simulink model "GolfSwing3D_InterfaceBlocks"  (R2024b)
settings: Solver=VariableStepAuto  StartTime=0.0  StopTime=StopTime  MaxStep=0.001  RelTol=1e-3
model workspace: external: MAT-File 3DModelInputs.mat (data not in the file)
undefined symbols (not defined in the file or in its folder): GripStrength, KillswitchFinalValue, KillswitchInitialValue, KillswitchStepTime, LeftLowerArmLength, PlaneTilt, RightLowerArmLength, UpperTorsoLength, X, Y, Z
libraries: nesl_utility x356, sm_lib x136, matrix_library x11, fl_lib x6, simulink x1
(part 4 of 13)

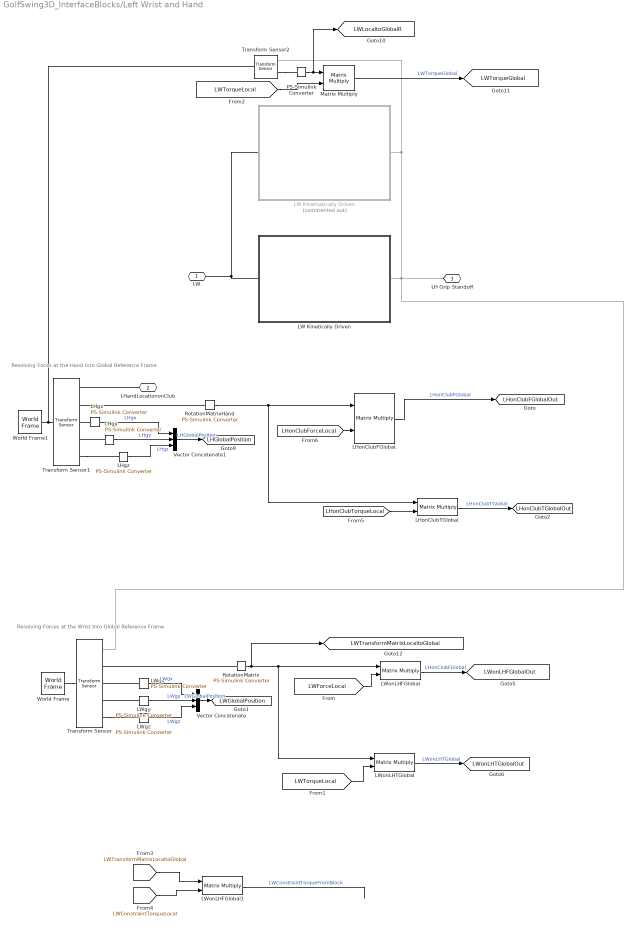
== system GolfSwing3D_InterfaceBlocks/Left Wrist and Hand ==
  note: Resolving Forces at the Wrist Into Global Reference Frame
  note: Resolving Foces at the Hand Into Global Reference Frame
  LHgx : nesl_utility/PS-Simulink Converter  PhysicalDomain=network_engine_domain  SubClassName=ps_output  LeftPortType=input  RightPortType=output  PseudoPeriodic=off  Frequencies=[]  VectorFormat=1-D array  Unit=inherit  AffineConversion=off
  LHgy : nesl_utility/PS-Simulink Converter  PhysicalDomain=network_engine_domain  SubClassName=ps_output  LeftPortType=input  RightPortType=output  PseudoPeriodic=off  Frequencies=[]  VectorFormat=1-D array  Unit=inherit  AffineConversion=off
  LHgz : nesl_utility/PS-Simulink Converter  PhysicalDomain=network_engine_domain  SubClassName=ps_output  LeftPortType=input  RightPortType=output  PseudoPeriodic=off  Frequencies=[]  VectorFormat=1-D array  Unit=inherit  AffineConversion=off
  LHonClubFGlobal. : Product  Multiplication=Matrix(*)
  LHonClubTGlobal. : Product  Multiplication=Matrix(*)
  LW Kinematically Driven : Subsystem  Commented=on
  LW Kinetically Driven : Subsystem
  LWgx : nesl_utility/PS-Simulink Converter  PhysicalDomain=network_engine_domain  SubClassName=ps_output  LeftPortType=input  RightPortType=output  PseudoPeriodic=off  Frequencies=[]  VectorFormat=1-D array  Unit=inherit  AffineConversion=off
  LWgy : nesl_utility/PS-Simulink Converter  PhysicalDomain=network_engine_domain  SubClassName=ps_output  LeftPortType=input  RightPortType=output  PseudoPeriodic=off  Frequencies=[]  VectorFormat=1-D array  Unit=inherit  AffineConversion=off
  LWgz : nesl_utility/PS-Simulink Converter  PhysicalDomain=network_engine_domain  SubClassName=ps_output  LeftPortType=input  RightPortType=output  PseudoPeriodic=off  Frequencies=[]  VectorFormat=1-D array  Unit=inherit  AffineConversion=off
  LWonLHFGlobal : Product  Multiplication=Matrix(*)
  LWonLHFGlobal1 : Product  Multiplication=Matrix(*)
  LWonLHTGlobal : Product  Multiplication=Matrix(*)
  Matrix Multiply : Product  Multiplication=Matrix(*)
  PS-Simulink Converter : nesl_utility/PS-Simulink Converter  PhysicalDomain=network_engine_domain  SubClassName=ps_output  LeftPortType=input  RightPortType=output  PseudoPeriodic=off  Frequencies=[]  VectorFormat=1-D array  Unit=inherit  AffineConversion=off
  RotationMatrix : nesl_utility/PS-Simulink Converter  PhysicalDomain=network_engine_domain  SubClassName=ps_output  LeftPortType=input  RightPortType=output  PseudoPeriodic=off  Frequencies=[]  VectorFormat=1-D array  Unit=inherit  AffineConversion=off
  RotationMatrixHand : nesl_utility/PS-Simulink Converter  PhysicalDomain=network_engine_domain  SubClassName=ps_output  LeftPortType=input  RightPortType=output  PseudoPeriodic=off  Frequencies=[]  VectorFormat=1-D array  Unit=inherit  AffineConversion=off
  Transform Sensor : sm_lib/Frames and Transforms/Transform Sensor  MeasurementFrame=World  RotationSequence=XYX  SenseAngle=off  SenseAxis=off  SenseQ=off  SenseR=on  SenseRotationSequence=off  SenseOmegaX=off  SenseOmegaY=off  SenseOmegaZ=off  SenseOmega=off  SenseQDot=off  SenseRDot=off  SenseRotationSequenceDot=off  SenseAlphaX=off  SenseAlphaY=off  SenseAlphaZ=off  SenseAlpha=off  SenseQDDot=off  SenseRDDot=off  SenseX=on  SenseY=on  SenseZ=on  SenseXYZ=off  SenseRad=off  SenseAzim=off  SenseDist=off  SenseInc=off  SenseXDot=off  SenseYDot=off  SenseZDot=off  SenseXYZDot=off  SenseRadDot=off  SenseAzimDot=off  SenseDistDot=off  SenseIncDot=off  SenseXDDot=off  SenseYDDot=off  SenseZDDot=off  SenseXYZDDot=off  SenseRadDDot=off  SenseAzimDDot=off  SenseDistDDot=off  SenseIncDDot=off
  Transform Sensor1 : sm_lib/Frames and Transforms/Transform Sensor  MeasurementFrame=World  RotationSequence=XYX  SenseAngle=off  SenseAxis=off  SenseQ=off  SenseR=on  SenseRotationSequence=off  SenseOmegaX=off  SenseOmegaY=off  SenseOmegaZ=off  SenseOmega=off  SenseQDot=off  SenseRDot=off  SenseRotationSequenceDot=off  SenseAlphaX=off  SenseAlphaY=off  SenseAlphaZ=off  SenseAlpha=off  SenseQDDot=off  SenseRDDot=off  SenseX=on  SenseY=on  SenseZ=on  SenseXYZ=off  SenseRad=off  SenseAzim=off  SenseDist=off  SenseInc=off  SenseXDot=off  SenseYDot=off  SenseZDot=off  SenseXYZDot=off  SenseRadDot=off  SenseAzimDot=off  SenseDistDot=off  SenseIncDot=off  SenseXDDot=off  SenseYDDot=off  SenseZDDot=off  SenseXYZDDot=off  SenseRadDDot=off  SenseAzimDDot=off  SenseDistDDot=off  SenseIncDDot=off
  Transform Sensor2 : sm_lib/Frames and Transforms/Transform Sensor  MeasurementFrame=World  RotationSequence=XYX  SenseAngle=off  SenseAxis=off  SenseQ=off  SenseR=on  SenseRotationSequence=off  SenseOmegaX=off  SenseOmegaY=off  SenseOmegaZ=off  SenseOmega=off  SenseQDot=off  SenseRDot=off  SenseRotationSequenceDot=off  SenseAlphaX=off  SenseAlphaY=off  SenseAlphaZ=off  SenseAlpha=off  SenseQDDot=off  SenseRDDot=off  SenseX=off  SenseY=off  SenseZ=off  SenseXYZ=off  SenseRad=off  SenseAzim=off  SenseDist=off  SenseInc=off  SenseXDot=off  SenseYDot=off  SenseZDot=off  SenseXYZDot=off  SenseRadDot=off  SenseAzimDot=off  SenseDistDot=off  SenseIncDot=off  SenseXDDot=off  SenseYDDot=off  SenseZDDot=off  SenseXYZDDot=off  SenseRadDDot=off  SenseAzimDDot=off  SenseDistDDot=off  SenseIncDDot=off
  Vector Concatenate : Concatenate  NumInputs=3
  Vector Concatenate1 : Concatenate  NumInputs=3
  World Frame : sm_lib/Frames and Transforms/World Frame
  World Frame1 : sm_lib/Frames and Transforms/World Frame
  LW : PMIOPort  Side=Left
  LHandLocationonClub : PMIOPort  Port=2  Side=Right
  LH Grip Standoff : PMIOPort  Port=3  Side=Right
  tag scope: LHGlobalPosition=global, LHonClubFGlobalOut=global, LHonClubTGlobalOut=global, LWGlobalPosition=global, LWLocaltoGlobalR=global, LWTorqueGlobal=global, LWTransformMatrixLocaltoGlobal=global, LWonLHFGlobalOut=global, LWonLHTGlobalOut=global
  wires:
  RotationMatrix/1 -> [LWTransformMatrixLocaltoGlobal], LWonLHFGlobal/1, LWonLHTGlobal/1
  LWonLHTGlobal/1 -> [LWonLHTGlobalOut]  "LWonLHTGlobal"
  LWonLHFGlobal/1 -> [LWonLHFGlobalOut]  "LHonClubFGlobal"
  LWgx/1 -> Vector Concatenate/1  "LWgx"
  LWgz/1 -> Vector Concatenate/3  "LWgz"
  Vector Concatenate/1 -> [LWGlobalPosition]  "LWGlobalPosition"
  LWgy/1 -> Vector Concatenate/2  "LWgy"
  [LHonClubTorqueLocal] -> LHonClubTGlobal./2
  LHgz/1 -> Vector Concatenate1/3  "LHgz"
  RotationMatrixHand/1 -> LHonClubTGlobal./1, LHonClubFGlobal./1
  LHgy/1 -> Vector Concatenate1/2  "LHgy"
  [LHonClubForceLocal] -> LHonClubFGlobal./2
  LHonClubTGlobal./1 -> [LHonClubTGlobalOut]  "LHonClubTGlobal"
  LHonClubFGlobal./1 -> [LHonClubFGlobalOut]  "LHonClubFGlobal"
  Vector Concatenate1/1 -> [LHGlobalPosition]  "LHGlobalPosition"
  LHgx/1 -> Vector Concatenate1/1  "LHgx"
  [LWForceLocal] -> LWonLHFGlobal/2
  [LWTorqueLocal] -> LWonLHTGlobal/2
  Matrix Multiply/1 -> [LWTorqueGlobal]  "LWTorqueGlobal"
  [LWTorqueLocal] -> Matrix Multiply/2
  PS-Simulink Converter/1 -> [LWLocaltoGlobalR], Matrix Multiply/1
  [LWTransformMatrixLocaltoGlobal] -> LWonLHFGlobal1/1
  [LWConstraintTorqueLocal] -> LWonLHFGlobal1/2
  LWonLHFGlobal1/1 -> ?  "LWConstraintTorqueFromBlock"
  connections:
  World Frame/RConn1 -- Transform Sensor/LConn1
  RotationMatrix/LConn1 -- Transform Sensor/RConn2
  LWgx/LConn1 -- Transform Sensor/RConn3
  LWgy/LConn1 -- Transform Sensor/RConn4
  Transform Sensor/RConn5 -- LWgz/LConn1
  Transform Sensor1/RConn5 -- LHgz/LConn1
  LHandLocationonClub/RConn1 -- Transform Sensor1/RConn1
  RotationMatrixHand/LConn1 -- Transform Sensor1/RConn2
  LHgy/LConn1 -- Transform Sensor1/RConn4
  World Frame1/RConn1 -- Transform Sensor2/LConn1 -- Transform Sensor1/LConn1
  LHgx/LConn1 -- Transform Sensor1/RConn3
  LW Kinematically Driven/RConn1 -- LW Kinetically Driven/RConn1 -- LH Grip Standoff/RConn1 -- Transform Sensor/RConn1 -- Transform Sensor2/RConn1
  LW Kinetically Driven/LConn1 -- LW Kinematically Driven/LConn1 -- LW/RConn1
  Transform Sensor2/RConn2 -- PS-Simulink Converter/LConn1

== system GolfSwing3D_InterfaceBlocks/Midpoint ==
  Hand Speed (mph) : Gain  Gain=2.23694
  MP MOF Global : matrix_library/Cross Product
  MP Unit Vector : MATLAB Function  TreatAsAtomicUnit=on  SystemSampleTime=0
  MPRVector : Sum  Inputs=+-
  MPUV : Mux  Inputs=3
  MPvx : nesl_utility/PS-Simulink Converter  PhysicalDomain=network_engine_domain  SubClassName=ps_output  LeftPortType=input  RightPortType=output  PseudoPeriodic=off  Frequencies=[]  VectorFormat=1-D array  Unit=inherit  AffineConversion=off
  MPvy : nesl_utility/PS-Simulink Converter  PhysicalDomain=network_engine_domain  SubClassName=ps_output  LeftPortType=input  RightPortType=output  PseudoPeriodic=off  Frequencies=[]  VectorFormat=1-D array  Unit=inherit  AffineConversion=off
  MPvz : nesl_utility/PS-Simulink Converter  PhysicalDomain=network_engine_domain  SubClassName=ps_output  LeftPortType=input  RightPortType=output  PseudoPeriodic=off  Frequencies=[]  VectorFormat=1-D array  Unit=inherit  AffineConversion=off
  MPx : nesl_utility/PS-Simulink Converter  PhysicalDomain=network_engine_domain  SubClassName=ps_output  LeftPortType=input  RightPortType=output  PseudoPeriodic=off  Frequencies=[]  VectorFormat=1-D array  Unit=inherit  AffineConversion=off
  MPy : nesl_utility/PS-Simulink Converter  PhysicalDomain=network_engine_domain  SubClassName=ps_output  LeftPortType=input  RightPortType=output  PseudoPeriodic=off  Frequencies=[]  VectorFormat=1-D array  Unit=inherit  AffineConversion=off
  MPz : nesl_utility/PS-Simulink Converter  PhysicalDomain=network_engine_domain  SubClassName=ps_output  LeftPortType=input  RightPortType=output  PseudoPeriodic=off  Frequencies=[]  VectorFormat=1-D array  Unit=inherit  AffineConversion=off
  MidpointAV : nesl_utility/PS-Simulink Converter  PhysicalDomain=network_engine_domain  SubClassName=ps_output  LeftPortType=input  RightPortType=output  PseudoPeriodic=off  Frequencies=[]  VectorFormat=1-D array  Unit=deg/s  AffineConversion=off
  Mux3 : Mux  Inputs=3
  Mux4 : Mux  Inputs=3
  Mux9 : Mux  Inputs=3
  Transform Sensor8 : sm_lib/Frames and Transforms/Transform Sensor  MeasurementFrame=World  RotationSequence=XYX  SenseAngle=off  SenseAxis=off  SenseQ=off  SenseR=off  SenseRotationSequence=off  SenseOmegaX=off  SenseOmegaY=off  SenseOmegaZ=off  SenseOmega=on  SenseQDot=off  SenseRDot=off  SenseRotationSequenceDot=off  SenseAlphaX=off  SenseAlphaY=off  SenseAlphaZ=off  SenseAlpha=off  SenseQDDot=off  SenseRDDot=off  SenseX=on  SenseY=on  SenseZ=on  SenseXYZ=off  SenseRad=off  SenseAzim=off  SenseDist=off  SenseInc=off  SenseXDot=on  SenseYDot=on  SenseZDot=on  SenseXYZDot=off  SenseRadDot=off  SenseAzimDot=off  SenseDistDot=off  SenseIncDot=off  SenseXDDot=off  SenseYDDot=off  SenseZDDot=off  SenseXYZDDot=off  SenseRadDDot=off  SenseAzimDDot=off  SenseDistDDot=off  SenseIncDDot=off
  Global Reference : PMIOPort  Side=Left
  MP : PMIOPort  Port=2  Side=Right
  tag scope: MPMOFonClubGlobal=global, MidpointUnitVector=global, MidpointVelocity=global
  wires:
  [ClubCOM] -> MPRVector/2
  MP Unit Vector/4(MPuvz) -> MPUV/3
  Mux4/1 -> [MidpointVelocity]  "MidpointVelocity"
  MPUV/1 -> [MidpointUnitVector]  "MidpointUnitVector"
  MPRVector/1 -> MP MOF Global/1
  MPvx/1 -> Mux9/1, MP Unit Vector/2(MPvx), Mux4/1  "MPvx"
  Mux9/1 -> MP Unit Vector/1(MPv)
  MP Unit Vector/1(MidHandSpeed) -> Hand Speed (mph)/1  "MidHandSpeed"
  MPvy/1 -> Mux9/2, MP Unit Vector/3(MPvy), Mux4/2  "MPvy"
  MPvz/1 -> Mux9/3, MP Unit Vector/4(MPvz), Mux4/3  "MPvz"
  MP Unit Vector/2(MPuvx) -> MPUV/1
  MPx/1 -> Mux3/1  "MPx"
  MP Unit Vector/3(MPuvy) -> MPUV/2
  MP MOF Global/1 -> [MPMOFonClubGlobal]  "MPMOFonClubGlobal"
  MPz/1 -> Mux3/3  "MPz"
  Mux3/1 -> MPRVector/1  "MidHandPosition"
  MPy/1 -> Mux3/2  "MPy"
  [TotalHandForceGlobal] -> MP MOF Global/2
  connections:
  Transform Sensor8/RConn1 -- MP/RConn1
  MPx/LConn1 -- Transform Sensor8/RConn3
  MidpointAV/LConn1 -- Transform Sensor8/RConn2
  MPvy/LConn1 -- Transform Sensor8/RConn7
  Global Reference/RConn1 -- Transform Sensor8/LConn1
  MPy/LConn1 -- Transform Sensor8/RConn4
  MPvx/LConn1 -- Transform Sensor8/RConn6
  MPz/LConn1 -- Transform Sensor8/RConn5
  MPvz/LConn1 -- Transform Sensor8/RConn8

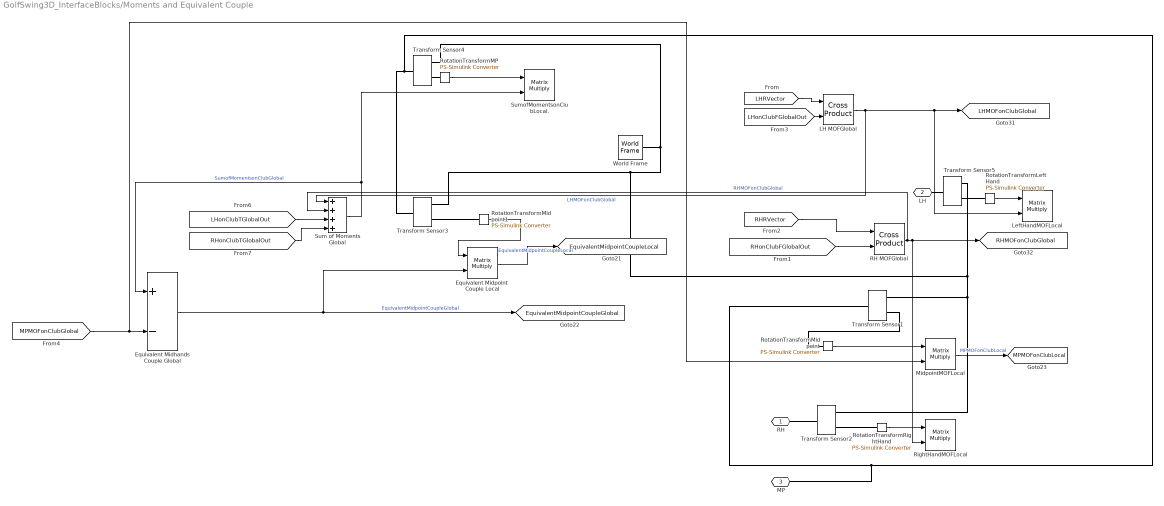
== system GolfSwing3D_InterfaceBlocks/Moments and Equivalent Couple ==
  Equivalent Midhands Couple Global : Sum  Inputs=+-
  Equivalent Midpoint Couple Local : Product  Multiplication=Matrix(*)
  LH MOFGlobal : matrix_library/Cross Product
  LeftHandMOFLocal : Product  Multiplication=Matrix(*)
  MidpointMOFLocal : Product  Multiplication=Matrix(*)
  RH MOFGlobal : matrix_library/Cross Product
  RightHandMOFLocal : Product  Multiplication=Matrix(*)
  RotationTransformLeftHand : nesl_utility/PS-Simulink Converter  PhysicalDomain=network_engine_domain  SubClassName=ps_output  LeftPortType=input  RightPortType=output  PseudoPeriodic=off  Frequencies=[]  VectorFormat=1-D array  Unit=inherit  AffineConversion=off
  RotationTransformMP : nesl_utility/PS-Simulink Converter  PhysicalDomain=network_engine_domain  SubClassName=ps_output  LeftPortType=input  RightPortType=output  PseudoPeriodic=off  Frequencies=[]  VectorFormat=1-D array  Unit=inherit  AffineConversion=off
  RotationTransformMidpoint : nesl_utility/PS-Simulink Converter  PhysicalDomain=network_engine_domain  SubClassName=ps_output  LeftPortType=input  RightPortType=output  PseudoPeriodic=off  Frequencies=[]  VectorFormat=1-D array  Unit=inherit  AffineConversion=off
  RotationTransformMidpoint1 : nesl_utility/PS-Simulink Converter  PhysicalDomain=network_engine_domain  SubClassName=ps_output  LeftPortType=input  RightPortType=output  PseudoPeriodic=off  Frequencies=[]  VectorFormat=1-D array  Unit=inherit  AffineConversion=off
  RotationTransformRightHand : nesl_utility/PS-Simulink Converter  PhysicalDomain=network_engine_domain  SubClassName=ps_output  LeftPortType=input  RightPortType=output  PseudoPeriodic=off  Frequencies=[]  VectorFormat=1-D array  Unit=inherit  AffineConversion=off
  Sum of Moments Global : Sum  Inputs=++++
  SumofMomentsonClubLocal. : Product  Multiplication=Matrix(*)
  Transform Sensor{1..5} (5 alike) : sm_lib/Frames and Transforms/Transform Sensor  MeasurementFrame=World  RotationSequence=XYX  SenseAngle=off  SenseAxis=off  SenseQ=off  SenseR=on  SenseRotationSequence=off  SenseOmegaX=off  SenseOmegaY=off  SenseOmegaZ=off  SenseOmega=off  SenseQDot=off  SenseRDot=off  SenseRotationSequenceDot=off  SenseAlphaX=off  SenseAlphaY=off  SenseAlphaZ=off  SenseAlpha=off  SenseQDDot=off  SenseRDDot=off  SenseX=off  SenseY=off  SenseZ=off  SenseXYZ=off  SenseRad=off  SenseAzim=off  SenseDist=off  SenseInc=off  SenseXDot=off  SenseYDot=off  SenseZDot=off  SenseXYZDot=off  SenseRadDot=off  SenseAzimDot=off  SenseDistDot=off  SenseIncDot=off  SenseXDDot=off  SenseYDDot=off  SenseZDDot=off  SenseXYZDDot=off  SenseRadDDot=off  SenseAzimDDot=off  SenseDistDDot=off  SenseIncDDot=off
  World Frame : sm_lib/Frames and Transforms/World Frame
  RH : PMIOPort  Side=Left
  LH : PMIOPort  Port=2  Side=Left
  MP : PMIOPort  Port=3  Side=Left
  tag scope: EquivalentMidpointCoupleGlobal=global, EquivalentMidpointCoupleLocal=global, LHMOFonClubGlobal=global, MPMOFonClubLocal=global, RHMOFonClubGlobal=global
  wires:
  [LHonClubFGlobalOut] -> LH MOFGlobal/2
  [RHonClubTGlobalOut] -> Sum of Moments Global/4
  Sum of Moments Global/1 -> Equivalent Midhands Couple Global/1, SumofMomentsonClubLocal./2  "SumofMomentsonClubGlobal"
  RH MOFGlobal/1 -> [RHMOFonClubGlobal], RightHandMOFLocal/2, Sum of Moments Global/2  "RHMOFonClubGlobal"
  [LHonClubTGlobalOut] -> Sum of Moments Global/3
  RotationTransformLeftHand/1 -> LeftHandMOFLocal/1
  [LHRVector] -> LH MOFGlobal/1
  Equivalent Midpoint Couple Local/1 -> [EquivalentMidpointCoupleLocal]  "EquivalentMidpointCoupleLocal"
  MidpointMOFLocal/1 -> [MPMOFonClubLocal]  "MPMOFonClubLocal"
  [MPMOFonClubGlobal] -> MidpointMOFLocal/2, Equivalent Midhands Couple Global/2
  LH MOFGlobal/1 -> LeftHandMOFLocal/2, [LHMOFonClubGlobal], Sum of Moments Global/1  "LHMOFonClubGlobal"
  RotationTransformMP/1 -> SumofMomentsonClubLocal./1
  RotationTransformMidpoint1/1 -> Equivalent Midpoint Couple Local/1
  Equivalent Midhands Couple Global/1 -> Equivalent Midpoint Couple Local/2, [EquivalentMidpointCoupleGlobal]  "EquivalentMidpointCoupleGlobal"
  RotationTransformMidpoint/1 -> MidpointMOFLocal/1
  RotationTransformRightHand/1 -> RightHandMOFLocal/1
  [RHonClubFGlobalOut] -> RH MOFGlobal/2
  [RHRVector] -> RH MOFGlobal/1
  connections:
  Transform Sensor1/LConn1 -- MP/RConn1 -- Transform Sensor3/LConn1 -- Transform Sensor4/LConn1
  World Frame/RConn1 -- Transform Sensor4/RConn1 -- Transform Sensor3/RConn1 -- Transform Sensor5/RConn1 -- Transform Sensor2/RConn1 -- Transform Sensor1/RConn1
  RotationTransformLeftHand/LConn1 -- Transform Sensor5/RConn2
  RotationTransformMidpoint1/LConn1 -- Transform Sensor3/RConn2
  RotationTransformMP/LConn1 -- Transform Sensor4/RConn2
  RH/RConn1 -- Transform Sensor2/LConn1
  RotationTransformMidpoint/LConn1 -- Transform Sensor1/RConn2
  RotationTransformRightHand/LConn1 -- Transform Sensor2/RConn2
  LH/RConn1 -- Transform Sensor5/LConn1

== system GolfSwing3D_InterfaceBlocks/RE Input Function ==
  Right Elbow Input Torque : MATLAB Function  TreatAsAtomicUnit=on  SystemSampleTime=0
  tag scope: FcnOutREAcceleration=global, FcnOutREPosition=global, FcnOutRETorque=global, FcnOutREVelocity=global
  wires:
  Right Elbow Input Torque/4(REAccelerationInput) -> [FcnOutREAcceleration]
  [Time] -> Right Elbow Input Torque/1(Time)
  Right Elbow Input Torque/1(JointTorqueRE) -> [FcnOutRETorque]  "RETorqueInput"
  Right Elbow Input Torque/2(REPositionInput) -> [FcnOutREPosition]
  Right Elbow Input Torque/3(REVelocityInput) -> [FcnOutREVelocity]
  [Killswitch] -> Right Elbow Input Torque/2(Killswitch)
  [REVelocity] -> Right Elbow Input Torque/4(REVelocity)
  [REPosition] -> Right Elbow Input Torque/3(REPosition)

== system GolfSwing3D_InterfaceBlocks/RF Input Function ==
  RF Input Torque : MATLAB Function  TreatAsAtomicUnit=on  SystemSampleTime=0
  tag scope: FcnOutRFAcceleration=global, FcnOutRFPosition=global, FcnOutRFTorque=global, FcnOutRFVelocity=global
  wires:
  RF Input Torque/1(JointTorqueRF) -> [FcnOutRFTorque]  "RFTorqueInput"
  [Time] -> RF Input Torque/1(Time)
  RF Input Torque/3(RFVelocityInput) -> [FcnOutRFVelocity]  "RFVelocity"
  [RFVelocity] -> RF Input Torque/4(RFVelocity)
  RF Input Torque/2(RFPositionInput) -> [FcnOutRFPosition]  "RFPosition"
  RF Input Torque/4(RFAccelerationInput) -> [FcnOutRFAcceleration]  "RFAcceleration"
  [RFPosition] -> RF Input Torque/3(RFPosition)
  [Killswitch] -> RF Input Torque/2(Killswitch)

== system GolfSwing3D_InterfaceBlocks/RS Input Function ==
  Right Shoulder Torque Output : MATLAB Function  TreatAsAtomicUnit=on  SystemSampleTime=0
  tag scope: FcnOutRSAccelerationX=global, FcnOutRSAccelerationY=global, FcnOutRSAccelerationZ=global, FcnOutRSPositionX=global, FcnOutRSPositionY=global, FcnOutRSPositionZ=global, FcnOutRSTorqueX=global, FcnOutRSTorqueY=global, FcnOutRSTorqueZ=global, FcnOutRSVelocityX=global, FcnOutRSVelocityY=global, FcnOutRSVelocityZ=global
  wires:
  Right Shoulder Torque Output/5(RSPositionInputY) -> [FcnOutRSPositionY]  "RSPositionInputY"
  [Killswitch] -> Right Shoulder Torque Output/2(Killswitch)
  Right Shoulder Torque Output/2(JointTorqueRSY) -> [FcnOutRSTorqueY]  "RSTorqueYInput"
  Right Shoulder Torque Output/11(RSAccelerationInputY) -> [FcnOutRSAccelerationY]  "RSAccelerationInputY"
  Right Shoulder Torque Output/12(RSAccelerationInputZ) -> [FcnOutRSAccelerationZ]  "RSAccelerationInputZ"
  Right Shoulder Torque Output/6(RSPositionInputZ) -> [FcnOutRSPositionZ]  "RSPositionInputZ"
  Right Shoulder Torque Output/10(RSAccelerationInputX) -> [FcnOutRSAccelerationX]  "RSAccelerationInputX"
  Right Shoulder Torque Output/8(RSVelocityInputY) -> [FcnOutRSVelocityY]  "RSVelocityInputY"
  [Time] -> Right Shoulder Torque Output/1(Time)
  Right Shoulder Torque Output/1(JointTorqueRSX) -> [FcnOutRSTorqueX]  "RSTorqueXInput"
  Right Shoulder Torque Output/4(RSPositionInputX) -> [FcnOutRSPositionX]  "RSPositionInputX"
  Right Shoulder Torque Output/9(RSVelocityInputZ) -> [FcnOutRSVelocityZ]  "RSVelocityInputZ"
  Right Shoulder Torque Output/7(RSVelocityInputX) -> [FcnOutRSVelocityX]  "RSVelocityInputX"
  Right Shoulder Torque Output/3(JointTorqueRSZ) -> [FcnOutRSTorqueZ]  "RSTorqueZInput"
  [RSVelocityZ] -> Right Shoulder Torque Output/8(RSVelocityZ)
  [RSVelocityY] -> Right Shoulder Torque Output/7(RSVelocityY)
  [RSVelocityX] -> Right Shoulder Torque Output/6(RSVelocityX)
  [RSPositionZ] -> Right Shoulder Torque Output/5(RSPositionZ)
  [RSPositionY] -> Right Shoulder Torque Output/4(RSPositionY)
  [RSPositionX] -> Right Shoulder Torque Output/3(RSPositionX)

== system GolfSwing3D_InterfaceBlocks/RScap Input Function ==
  RScap Torque : MATLAB Function  TreatAsAtomicUnit=on  SystemSampleTime=0
  tag scope: FcnOutRScapAccelerationX=global, FcnOutRScapAccelerationY=global, FcnOutRScapPositionX=global, FcnOutRScapPositionY=global, FcnOutRScapTorqueX=global, FcnOutRScapTorqueY=global, FcnOutRScapVelocityX=global, FcnOutRScapVelocityY=global
  wires:
  RScap Torque/3(RScapPositionInputX) -> [FcnOutRScapPositionX]
  RScap Torque/1(JointTorqueRScapX) -> [FcnOutRScapTorqueX]  "RScapTorqueXInput"
  RScap Torque/5(RScapVelocityInputX) -> [FcnOutRScapVelocityX]
  [Time] -> RScap Torque/1(Time)
  RScap Torque/2(JointTorqueRScapY) -> [FcnOutRScapTorqueY]  "RScapTorqueYInput"
  [Killswitch] -> RScap Torque/2(Killswitch)
  RScap Torque/6(RScapVelocityInputY) -> [FcnOutRScapVelocityY]
  RScap Torque/4(RScapPositionInputY) -> [FcnOutRScapPositionY]
  [RScapPositionX] -> RScap Torque/3(RScapPositionX)
  [RScapPositionY] -> RScap Torque/4(RScapPositionY)
  RScap Torque/8(RScapAccelerationInputY) -> [FcnOutRScapAccelerationY]
  RScap Torque/7(RScapAccelerationInputX) -> [FcnOutRScapAccelerationX]
  [RScapVelocityY] -> RScap Torque/6(RScapVelocityY)
  [RScapVelocityX] -> RScap Torque/5(RScapVelocityX)

== system GolfSwing3D_InterfaceBlocks/RW Input Function ==
  Right Wrist Torque : MATLAB Function  TreatAsAtomicUnit=on  SystemSampleTime=0
  RWJointTorqueInputGlobal : Outport  PortDimensions=3
  RWConstraintTorque : Outport  Port=2  PortDimensions=3
  tag scope: FcnOutRWAccelerationX=global, FcnOutRWAccelerationY=global, FcnOutRWPositionX=global, FcnOutRWPositionY=global, FcnOutRWTorqueX=global, FcnOutRWTorqueY=global, FcnOutRWVelocityX=global, FcnOutRWVelocityY=global, RWConstraintTorque=global, RWJointTorqueInputGlobal=global
  wires:
  Right Wrist Torque/2(JointTorqueRWY) -> [FcnOutRWTorqueY]  "RWTorqueYInput"
  Right Wrist Torque/4(RWPositionInputY) -> [FcnOutRWPositionY]
  Right Wrist Torque/5(RWVelocityInputX) -> [FcnOutRWVelocityX]
  Right Wrist Torque/3(RWPositionInputX) -> [FcnOutRWPositionX]
  Right Wrist Torque/7(RWAccelerationInputX) -> [FcnOutRWAccelerationX]
  Right Wrist Torque/6(RWVelocityInputY) -> [FcnOutRWVelocityY]
  Right Wrist Torque/8(RWAccelerationInputY) -> [FcnOutRWAccelerationY]
  [Killswitch] -> Right Wrist Torque/2(Killswitch)
  [Time] -> Right Wrist Torque/1(Time)
  Right Wrist Torque/1(JointTorqueRWX) -> [FcnOutRWTorqueX]  "RWTorqueXInput"
  [RWPositionX] -> Right Wrist Torque/3(RWPositionX)
  [RWPositionY] -> Right Wrist Torque/4(RWPositionY)
  [RWVelocityX] -> Right Wrist Torque/5(RWVelocityX)
  [RWVelocityY] -> Right Wrist Torque/6(RWVelocityY)
  [RWLocaltoGlobalR] -> Right Wrist Torque/7(RWLocaltoGlobalR)
  [RWTorqueGlobal] -> Right Wrist Torque/8(RWTorqueGlobal)
  Right Wrist Torque/10(RWConstraintTorque) -> RWConstraintTorque/1, [RWConstraintTorque]  "RWConstraintTorque"
  Right Wrist Torque/9(RWJointTorqueInputGlobal) -> RWJointTorqueInputGlobal/1, [RWJointTorqueInputGlobal]  "RWJointTorqueInputGlobal"

== system GolfSwing3D_InterfaceBlocks/Right Elbow Joint ==
  note: REGlobal
  Dot Product1 : DotProduct  OutDataTypeStr=Inherit: Inherit via internal rule
  Dot Product3 : DotProduct  OutDataTypeStr=Inherit: Inherit via internal rule
  RArmonRFoearmTGlobal : Product  Multiplication=Matrix(*)
  RArmonRForearmFGlobal : Product  Multiplication=Matrix(*)
  RArmonRForearmFLocal : nesl_utility/PS-Simulink Converter  PhysicalDomain=network_engine_domain  SubClassName=ps_output  LeftPortType=input  RightPortType=output  PseudoPeriodic=off  Frequencies=[]  VectorFormat=1-D array  Unit=inherit  AffineConversion=off
  RArmonRForearmTLocal : nesl_utility/PS-Simulink Converter  PhysicalDomain=network_engine_domain  SubClassName=ps_output  LeftPortType=input  RightPortType=output  PseudoPeriodic=off  Frequencies=[]  VectorFormat=1-D array  Unit=inherit  AffineConversion=off
  RE Kinematically Driven : Subsystem  Commented=on
  RE Kinetically Driven : Subsystem
  REAV : nesl_utility/PS-Simulink Converter  PhysicalDomain=network_engine_domain  SubClassName=ps_output  LeftPortType=input  RightPortType=output  PseudoPeriodic=off  Frequencies=[]  VectorFormat=1-D array  Unit=inherit  AffineConversion=off
  REAngularWorkonForearm : Integrator
  REGlobalPosition : nesl_utility/PS-Simulink Converter  PhysicalDomain=network_engine_domain  SubClassName=ps_output  LeftPortType=input  RightPortType=output  PseudoPeriodic=off  Frequencies=[]  VectorFormat=1-D array  Unit=inherit  AffineConversion=off
  REGlobalVelocity : nesl_utility/PS-Simulink Converter  PhysicalDomain=network_engine_domain  SubClassName=ps_output  LeftPortType=input  RightPortType=output  PseudoPeriodic=off  Frequencies=[]  VectorFormat=1-D array  Unit=inherit  AffineConversion=off
  RELinearImpulseonForearm : Integrator
  RELinearWorkonForearm : Integrator
  REvGlobal : nesl_utility/PS-Simulink Converter  PhysicalDomain=network_engine_domain  SubClassName=ps_output  LeftPortType=input  RightPortType=output  PseudoPeriodic=off  Frequencies=[]  VectorFormat=1-D array  Unit=inherit  AffineConversion=off
  REx : nesl_utility/PS-Simulink Converter  PhysicalDomain=network_engine_domain  SubClassName=ps_output  LeftPortType=input  RightPortType=output  PseudoPeriodic=off  Frequencies=[]  VectorFormat=1-D array  Unit=inherit  AffineConversion=off
  REy : nesl_utility/PS-Simulink Converter  PhysicalDomain=network_engine_domain  SubClassName=ps_output  LeftPortType=input  RightPortType=output  PseudoPeriodic=off  Frequencies=[]  VectorFormat=1-D array  Unit=inherit  AffineConversion=off
  REz : nesl_utility/PS-Simulink Converter  PhysicalDomain=network_engine_domain  SubClassName=ps_output  LeftPortType=input  RightPortType=output  PseudoPeriodic=off  Frequencies=[]  VectorFormat=1-D array  Unit=inherit  AffineConversion=off
  RotationMatrix : nesl_utility/PS-Simulink Converter  PhysicalDomain=network_engine_domain  SubClassName=ps_output  LeftPortType=input  RightPortType=output  PseudoPeriodic=off  Frequencies=[]  VectorFormat=1-D array  Unit=inherit  AffineConversion=off
  Spherical Solid : sm_lib/Body Elements/Spherical Solid  SphereRadius=1.75  SphereRadiusUnits=in  ExportEntireGeometry=off  InertiaType=CalculateFromGeometry  BasedOnType=Density  Density=0  DensityUnits=kg/m^3  Mass=1  MassUnits=kg  CenterOfMass=[0 0 0]  CenterOfMassUnits=m  MomentsOfInertia=[1 1 1]  MomentsOfInertiaUnits=kg*m^2  ProductsOfInertia=[0 0 0]  ProductsOfInertiaUnits=kg*m^2  GraphicType=FromGeometry  MarkerShape=Sphere  MarkerSize=10  GraphicVisPropType=SimpleVisualProperties  GraphicDiffuseColor=[1.0 0.8 0.4]  GraphicOpacity=1  GraphicSpecularColor=[0.5 0.5 0.5 1.0]  GraphicAmbientColor=[0.15 0.15 0.15 1.0]  GraphicEmissiveColor=[0.0 0.0 0.0 1.0]  GraphicShininess=75  DoExposeReferenceFrame=on  SerializedFrames=<Frames/>
  Transform Sensor : sm_lib/Frames and Transforms/Transform Sensor  MeasurementFrame=World  RotationSequence=XYX  SenseAngle=off  SenseAxis=off  SenseQ=off  SenseR=on  SenseRotationSequence=off  SenseOmegaX=off  SenseOmegaY=off  SenseOmegaZ=off  SenseOmega=off  SenseQDot=off  SenseRDot=off  SenseRotationSequenceDot=off  SenseAlphaX=off  SenseAlphaY=off  SenseAlphaZ=off  SenseAlpha=off  SenseQDDot=off  SenseRDDot=off  SenseX=off  SenseY=off  SenseZ=off  SenseXYZ=on  SenseRad=off  SenseAzim=off  SenseDist=off  SenseInc=off  SenseXDot=off  SenseYDot=off  SenseZDot=off  SenseXYZDot=on  SenseRadDot=off  SenseAzimDot=off  SenseDistDot=off  SenseIncDot=off  SenseXDDot=off  SenseYDDot=off  SenseZDDot=off  SenseXYZDDot=off  SenseRadDDot=off  SenseAzimDDot=off  SenseDistDDot=off  SenseIncDDot=off
  Transform Sensor1 : sm_lib/Frames and Transforms/Transform Sensor  MeasurementFrame=World  RotationSequence=XYX  SenseAngle=off  SenseAxis=off  SenseQ=off  SenseR=off  SenseRotationSequence=off  SenseOmegaX=off  SenseOmegaY=off  SenseOmegaZ=off  SenseOmega=on  SenseQDot=off  SenseRDot=off  SenseRotationSequenceDot=off  SenseAlphaX=off  SenseAlphaY=off  SenseAlphaZ=off  SenseAlpha=off  SenseQDDot=off  SenseRDDot=off  SenseX=on  SenseY=on  SenseZ=on  SenseXYZ=off  SenseRad=off  SenseAzim=off  SenseDist=off  SenseInc=off  SenseXDot=off  SenseYDot=off  SenseZDot=off  SenseXYZDot=on  SenseRadDot=off  SenseAzimDot=off  SenseDistDot=off  SenseIncDot=off  SenseXDDot=off  SenseYDDot=off  SenseZDDot=off  SenseXYZDDot=off  SenseRadDDot=off  SenseAzimDDot=off  SenseDistDDot=off  SenseIncDDot=off
  World Frame : sm_lib/Frames and Transforms/World Frame
  Bottom of Right Arm : PMIOPort  Side=Left
  Top of Right Forearm : PMIOPort  Port=2  Side=Right
  tag scope: RArmonRForearmFGlobalOut=global, RArmonRForearmTGlobalOut=global, REGlobalPosition=global, REGlobalVelocity=global
  wires:
  RArmonRForearmFLocal/1 -> RArmonRForearmFGlobal/2
  RotationMatrix/1 -> RArmonRForearmFGlobal/1, RArmonRFoearmTGlobal/1
  RArmonRForearmTLocal/1 -> RArmonRFoearmTGlobal/2
  RArmonRForearmFGlobal/1 -> [RArmonRForearmFGlobalOut], Dot Product1/1, RELinearImpulseonForearm/1  "RArmonRForearmFGlobal"
  RArmonRFoearmTGlobal/1 -> [RArmonRForearmTGlobalOut], Dot Product3/1  "RArmonRForearmTGlobal"
  Dot Product3/1 -> REAngularWorkonForearm/1  "REonForearmAngularPower"
  Dot Product1/1 -> RELinearWorkonForearm/1  "REonForearmLinearPower"
  REvGlobal/1 -> Dot Product1/2  "REVGlobal"
  REAV/1 -> Dot Product3/2  "REAVGlobal"
  REGlobalPosition/1 -> [REGlobalPosition]  "REGlobalPosition"
  REGlobalVelocity/1 -> [REGlobalVelocity]  "REGlobalVelocity"
  connections:
  World Frame/RConn1 -- Transform Sensor1/LConn1 -- Transform Sensor/LConn1
  REGlobalVelocity/LConn1 -- Transform Sensor/RConn4
  RotationMatrix/LConn1 -- Transform Sensor/RConn2
  REvGlobal/LConn1 -- Transform Sensor1/RConn6
  REAV/LConn1 -- Transform Sensor1/RConn2
  REz/LConn1 -- Transform Sensor1/RConn5
  REy/LConn1 -- Transform Sensor1/RConn4
  REx/LConn1 -- Transform Sensor1/RConn3
  Transform Sensor1/RConn1 -- RE Kinetically Driven/LConn1 -- Bottom of Right Arm/RConn1 -- RE Kinematically Driven/LConn1 -- Spherical Solid/RConn1
  Top of Right Forearm/RConn1 -- Transform Sensor/RConn1 -- RE Kinetically Driven/RConn1 -- RE Kinematically Driven/RConn1
  RArmonRForearmFLocal/LConn1 -- RE Kinetically Driven/RConn2
  RE Kinetically Driven/RConn3 -- RArmonRForearmTLocal/LConn1
  REGlobalPosition/LConn1 -- Transform Sensor/RConn3

== system GolfSwing3D_InterfaceBlocks/Right Forearm ==
  Right Forearm : Subsystem
  Right Forearm MOF : Subsystem  Commented=on
  Right Elbow : PMIOPort  Side=Left
  Right Wrist : PMIOPort  Port=2  Side=Right
  connections:
  Right Forearm/RConn1 -- Right Wrist/RConn1
  Right Forearm/LConn1 -- Right Elbow/RConn1 -- Right Forearm MOF/LConn1

== system GolfSwing3D_InterfaceBlocks/Right Hand ==
  Mux10 : Mux  Inputs=3
  Mux5 : Mux  Inputs=3
  Mux6 : Mux  Inputs=3
  RHRVector : Sum  Inputs=+-
  RHvx : nesl_utility/PS-Simulink Converter  PhysicalDomain=network_engine_domain  SubClassName=ps_output  LeftPortType=input  RightPortType=output  PseudoPeriodic=off  Frequencies=[]  VectorFormat=1-D array  Unit=inherit  AffineConversion=off
  RHvy : nesl_utility/PS-Simulink Converter  PhysicalDomain=network_engine_domain  SubClassName=ps_output  LeftPortType=input  RightPortType=output  PseudoPeriodic=off  Frequencies=[]  VectorFormat=1-D array  Unit=inherit  AffineConversion=off
  RHvz : nesl_utility/PS-Simulink Converter  PhysicalDomain=network_engine_domain  SubClassName=ps_output  LeftPortType=input  RightPortType=output  PseudoPeriodic=off  Frequencies=[]  VectorFormat=1-D array  Unit=inherit  AffineConversion=off
  RHx : nesl_utility/PS-Simulink Converter  PhysicalDomain=network_engine_domain  SubClassName=ps_output  LeftPortType=input  RightPortType=output  PseudoPeriodic=off  Frequencies=[]  VectorFormat=1-D array  Unit=inherit  AffineConversion=off
  RHy : nesl_utility/PS-Simulink Converter  PhysicalDomain=network_engine_domain  SubClassName=ps_output  LeftPortType=input  RightPortType=output  PseudoPeriodic=off  Frequencies=[]  VectorFormat=1-D array  Unit=inherit  AffineConversion=off
  RHz : nesl_utility/PS-Simulink Converter  PhysicalDomain=network_engine_domain  SubClassName=ps_output  LeftPortType=input  RightPortType=output  PseudoPeriodic=off  Frequencies=[]  VectorFormat=1-D array  Unit=inherit  AffineConversion=off
  RW Unit Vector : MATLAB Function  TreatAsAtomicUnit=on  SystemSampleTime=0
  RWAV : nesl_utility/PS-Simulink Converter  PhysicalDomain=network_engine_domain  SubClassName=ps_output  LeftPortType=input  RightPortType=output  PseudoPeriodic=off  Frequencies=[]  VectorFormat=1-D array  Unit=deg/s  AffineConversion=off
  RightHandPathUnitVector : Mux  Inputs=3
  Transform Sensor9 : sm_lib/Frames and Transforms/Transform Sensor  MeasurementFrame=World  RotationSequence=XYX  SenseAngle=off  SenseAxis=off  SenseQ=off  SenseR=off  SenseRotationSequence=off  SenseOmegaX=off  SenseOmegaY=off  SenseOmegaZ=off  SenseOmega=on  SenseQDot=off  SenseRDot=off  SenseRotationSequenceDot=off  SenseAlphaX=off  SenseAlphaY=off  SenseAlphaZ=off  SenseAlpha=off  SenseQDDot=off  SenseRDDot=off  SenseX=on  SenseY=on  SenseZ=on  SenseXYZ=off  SenseRad=off  SenseAzim=off  SenseDist=off  SenseInc=off  SenseXDot=on  SenseYDot=on  SenseZDot=on  SenseXYZDot=off  SenseRadDot=off  SenseAzimDot=off  SenseDistDot=off  SenseIncDot=off  SenseXDDot=off  SenseYDDot=off  SenseZDDot=off  SenseXYZDDot=off  SenseRadDDot=off  SenseAzimDDot=off  SenseDistDDot=off  SenseIncDDot=off
  Global Reference : PMIOPort  Side=Left
  RH : PMIOPort  Port=2  Side=Right
  tag scope: RHAVGlobal=global, RHPathUV=global, RHRVector=global, RHVGlobal=global
  wires:
  Mux10/1 -> RW Unit Vector/1(RWv)
  RHvx/1 -> RW Unit Vector/2(RWvx), Mux10/1, Mux6/1  "RHvx"
  RW Unit Vector/4(RWuvz) -> RightHandPathUnitVector/3
  RHvz/1 -> RW Unit Vector/4(RWvz), Mux10/3, Mux6/3  "RHvz"
  RightHandPathUnitVector/1 -> [RHPathUV]  "RHPathUV"
  RHvy/1 -> Mux6/2, Mux10/2, RW Unit Vector/3(RWvy)  "RHvy"
  RHRVector/1 -> [RHRVector]
  RHx/1 -> Mux5/1  "RHx"
  RW Unit Vector/3(RWuvy) -> RightHandPathUnitVector/2
  RW Unit Vector/2(RWuvx) -> RightHandPathUnitVector/1
  RWAV/1 -> [RHAVGlobal]  "RHAVGlobal"
  Mux5/1 -> RHRVector/1  "RightHandPosition"
  RHy/1 -> Mux5/2  "RHy"
  Mux6/1 -> [RHVGlobal]  "RHVGlobal"
  RHz/1 -> Mux5/3  "RHz"
  [ClubCOM] -> RHRVector/2
  connections:
  RWAV/LConn1 -- Transform Sensor9/RConn2
  Transform Sensor9/LConn1 -- Global Reference/RConn1
  RHy/LConn1 -- Transform Sensor9/RConn4
  RHvy/LConn1 -- Transform Sensor9/RConn7
  RHvx/LConn1 -- Transform Sensor9/RConn6
  RHvz/LConn1 -- Transform Sensor9/RConn8
  RHz/LConn1 -- Transform Sensor9/RConn5
  Transform Sensor9/RConn1 -- RH/RConn1
  RHx/LConn1 -- Transform Sensor9/RConn3

== system GolfSwing3D_InterfaceBlocks/Right Scapula Joint ==
  RScap Kinematically Driven : Subsystem  Commented=on
  RScap Kinetically Driven : Subsystem
  COMRodTop : PMIOPort  Side=Left
  Hub : PMIOPort  Port=2  Side=Right
  connections:
  Hub/RConn1 -- RScap Kinetically Driven/RConn1 -- RScap Kinematically Driven/RConn1
  RScap Kinematically Driven/LConn1 -- COMRodTop/RConn1 -- RScap Kinetically Driven/LConn1

== system GolfSwing3D_InterfaceBlocks/Right Shoulder Joint ==
  note: RSGlobal
  Dot Product1 : DotProduct  OutDataTypeStr=Inherit: Inherit via internal rule
  Dot Product2 : DotProduct  OutDataTypeStr=Inherit: Inherit via internal rule
  RS Kinematically Driven : Subsystem  Commented=on
  RS Kinetically Driven : Subsystem
  RSAV : nesl_utility/PS-Simulink Converter  PhysicalDomain=network_engine_domain  SubClassName=ps_output  LeftPortType=input  RightPortType=output  PseudoPeriodic=off  Frequencies=[]  VectorFormat=1-D array  Unit=deg/s  AffineConversion=off
  RSAngularWorkonArm : Integrator
  RSGlobalPosition : nesl_utility/PS-Simulink Converter  PhysicalDomain=network_engine_domain  SubClassName=ps_output  LeftPortType=input  RightPortType=output  PseudoPeriodic=off  Frequencies=[]  VectorFormat=1-D array  Unit=inherit  AffineConversion=off
  RSLinearImpulseonArm : Integrator
  RSLinearWorkonArm : Integrator
  RSonRArmFGlob : Product  Multiplication=Matrix(*)
  RSonRArmLocalForce : nesl_utility/PS-Simulink Converter  PhysicalDomain=network_engine_domain  SubClassName=ps_output  LeftPortType=input  RightPortType=output  PseudoPeriodic=off  Frequencies=[]  VectorFormat=1-D array  Unit=inherit  AffineConversion=off
  RSonRArmLocalTorque : nesl_utility/PS-Simulink Converter  PhysicalDomain=network_engine_domain  SubClassName=ps_output  LeftPortType=input  RightPortType=output  PseudoPeriodic=off  Frequencies=[]  VectorFormat=1-D array  Unit=inherit  AffineConversion=off
  RSonRArmTGlobal : Product  Multiplication=Matrix(*)
  RSvGlobal : nesl_utility/PS-Simulink Converter  PhysicalDomain=network_engine_domain  SubClassName=ps_output  LeftPortType=input  RightPortType=output  PseudoPeriodic=off  Frequencies=[]  VectorFormat=1-D array  Unit=inherit  AffineConversion=off
  RotationMatrix : nesl_utility/PS-Simulink Converter  PhysicalDomain=network_engine_domain  SubClassName=ps_output  LeftPortType=input  RightPortType=output  PseudoPeriodic=off  Frequencies=[]  VectorFormat=1-D array  Unit=inherit  AffineConversion=off
  Spherical Solid : sm_lib/Body Elements/Spherical Solid  SphereRadius=1.75  SphereRadiusUnits=in  ExportEntireGeometry=off  InertiaType=CalculateFromGeometry  BasedOnType=Density  Density=0  DensityUnits=kg/m^3  Mass=1  MassUnits=kg  CenterOfMass=[0 0 0]  CenterOfMassUnits=m  MomentsOfInertia=[1 1 1]  MomentsOfInertiaUnits=kg*m^2  ProductsOfInertia=[0 0 0]  ProductsOfInertiaUnits=kg*m^2  GraphicType=FromGeometry  MarkerShape=Sphere  MarkerSize=10  GraphicVisPropType=SimpleVisualProperties  GraphicDiffuseColor=[0.2 0.2 1.0]  GraphicOpacity=1  GraphicSpecularColor=[0.5 0.5 0.5 1.0]  GraphicAmbientColor=[0.15 0.15 0.15 1.0]  GraphicEmissiveColor=[0.0 0.0 0.0 1.0]  GraphicShininess=75  DoExposeReferenceFrame=on  SerializedFrames=<Frames/>
  Transform Sensor1 : sm_lib/Frames and Transforms/Transform Sensor  MeasurementFrame=World  RotationSequence=XYX  SenseAngle=off  SenseAxis=off  SenseQ=off  SenseR=on  SenseRotationSequence=off  SenseOmegaX=off  SenseOmegaY=off  SenseOmegaZ=off  SenseOmega=on  SenseQDot=off  SenseRDot=off  SenseRotationSequenceDot=off  SenseAlphaX=off  SenseAlphaY=off  SenseAlphaZ=off  SenseAlpha=off  SenseQDDot=off  SenseRDDot=off  SenseX=off  SenseY=off  SenseZ=off  SenseXYZ=on  SenseRad=off  SenseAzim=off  SenseDist=off  SenseInc=off  SenseXDot=off  SenseYDot=off  SenseZDot=off  SenseXYZDot=on  SenseRadDot=off  SenseAzimDot=off  SenseDistDot=off  SenseIncDot=off  SenseXDDot=off  SenseYDDot=off  SenseZDDot=off  SenseXYZDDot=off  SenseRadDDot=off  SenseAzimDDot=off  SenseDistDDot=off  SenseIncDDot=off
  World Frame : sm_lib/Frames and Transforms/World Frame
  Right Shoulder : PMIOPort  Side=Left
  Top of Right Arm : PMIOPort  Port=2  Side=Right
  tag scope: RSGlobalPosition=global, RSonRArmFGlobalOut=global, RSonRArmTGlobalOut=global
  wires:
  RotationMatrix/1 -> RSonRArmFGlob/1, RSonRArmTGlobal/1
  RSonRArmLocalForce/1 -> RSonRArmFGlob/2
  RSonRArmLocalTorque/1 -> RSonRArmTGlobal/2
  RSonRArmTGlobal/1 -> Dot Product2/1, [RSonRArmTGlobalOut]  "RSonRArmTGlobal"
  RSGlobalPosition/1 -> [RSGlobalPosition]  "RSGlobalPosition"
  Dot Product1/1 -> RSLinearWorkonArm/1  "RSonArmLinearPower"
  Dot Product2/1 -> RSAngularWorkonArm/1  "RSonArmAngularPower"
  RSonRArmFGlob/1 -> RSLinearImpulseonArm/1, Dot Product1/1, [RSonRArmFGlobalOut]  "RSonRArmFGlobal"
  RSvGlobal/1 -> Dot Product1/2  "RSVGlobal"
  RSAV/1 -> Dot Product2/2  "RSAVGlobal"
  connections:
  Spherical Solid/RConn1 -- RS Kinetically Driven/LConn1 -- Top of Right Arm/RConn1 -- RS Kinematically Driven/LConn1 -- Transform Sensor1/RConn1
  RotationMatrix/LConn1 -- Transform Sensor1/RConn2
  Transform Sensor1/LConn1 -- World Frame/RConn1
  Transform Sensor1/RConn5 -- RSvGlobal/LConn1
  RSAV/LConn1 -- Transform Sensor1/RConn3
  RS Kinematically Driven/RConn1 -- Right Shoulder/RConn1 -- RS Kinetically Driven/RConn1
  RSonRArmLocalForce/LConn1 -- RS Kinetically Driven/RConn2
  RSonRArmLocalTorque/LConn1 -- RS Kinetically Driven/RConn3
  RSGlobalPosition/LConn1 -- Transform Sensor1/RConn4

== system GolfSwing3D_InterfaceBlocks/Right Upper Arm ==
  Cylindrical Solid3 : sm_lib/Body Elements/Cylindrical Solid  CylinderRadius=1.75  CylinderRadiusUnits=in  CylinderLength=12  CylinderLengthUnits=in  ExportEntireGeometry=off  InertiaType=CalculateFromGeometry  BasedOnType=Mass  Density=1000  DensityUnits=kg/m^3  Mass=5  MassUnits=lbm  CenterOfMass=[0 0 0]  CenterOfMassUnits=m  MomentsOfInertia=[1 1 1]  MomentsOfInertiaUnits=kg*m^2  ProductsOfInertia=[0 0 0]  ProductsOfInertiaUnits=kg*m^2  GraphicType=FromGeometry  MarkerShape=Sphere  MarkerSize=10  GraphicVisPropType=SimpleVisualProperties  GraphicDiffuseColor=[0.2 0.2 1.0]  GraphicOpacity=1.0  GraphicSpecularColor=[0.5 0.5 0.5 1.0]  GraphicAmbientColor=[0.15 0.15 0.15 1.0]  GraphicEmissiveColor=[0.0 0.0 0.0 1.0]  GraphicShininess=75  DoExposeReferenceFrame=off  SerializedFrames=<Frames><Frame><Id>Frame1</Id><Value><Name>Top of Right Arm</Name><Origin><Source>GeometricFeature</Source><FeatureName>top curve</FeatureName></Origin><PrimaryAxis><DefinedDirection>-X</DefinedDirection><Source>ReferenceFrame</Source><SourceDirection>+Z</SourceDirection><FeatureName></FeatureName></PrimaryAxis><SecondaryAxis><DefinedDirection>+Y</DefinedDirection><Source>ReferenceFrame</Source><SourceDirection>+X</SourceDirection><FeatureName></FeatureName></SecondaryAxis></Value></Frame><Frame><Id>Frame2</Id><Value><Name>Bottom of Right Arm</Name><Origin><Source>GeometricFeature</Source><FeatureName>bottom curve</FeatureName></Origin><PrimaryAxis><DefinedDirection>-X</DefinedDirection><Source>ReferenceFrame</Source><SourceDirection>+Z</SourceDirection><FeatureName></FeatureName></PrimaryAxis><SecondaryAxis><DefinedDirection>+Z</DefinedDirection><Source>ReferenceFrame</Source><SourceDirection>-X</SourceDirection><FeatureName></FeatureName></SecondaryAxis></Value></Frame></Frames>
  Right Upper Arm MOF : Subsystem  Commented=on
  RightUpper  Arm : PMIOPort  Side=Left
  Right Elbow : PMIOPort  Port=2  Side=Right
  connections:
  Right Upper Arm MOF/LConn1 -- RightUpper  Arm/RConn1 -- Cylindrical Solid3/LConn1
  Cylindrical Solid3/RConn1 -- Right Elbow/RConn1

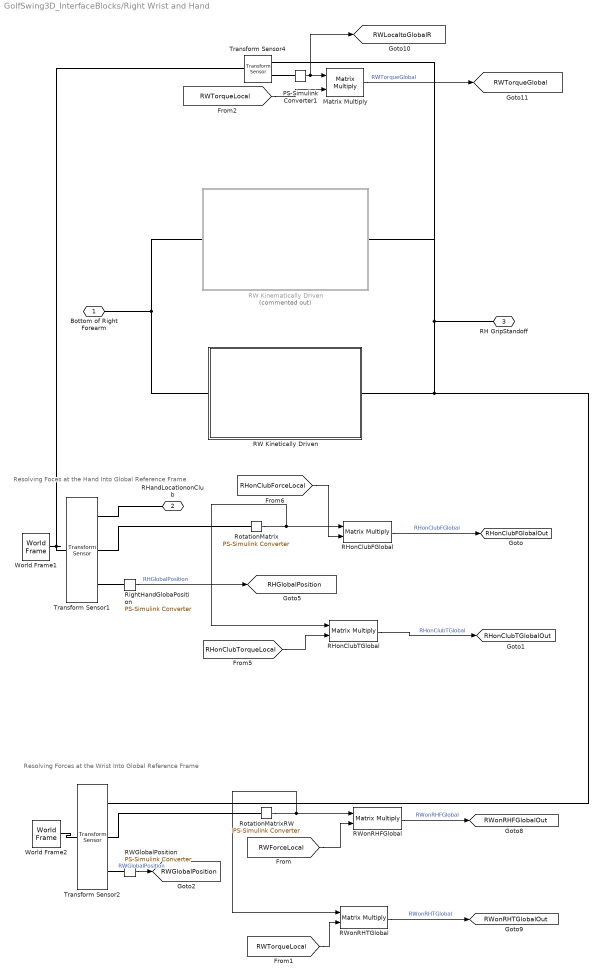
== system GolfSwing3D_InterfaceBlocks/Right Wrist and Hand ==
  note: Resolving Foces at the Hand Into Global Reference Frame
  note: Resolving Forces at the Wrist Into Global Reference Frame
  Matrix Multiply : Product  Multiplication=Matrix(*)
  PS-Simulink Converter1 : nesl_utility/PS-Simulink Converter  PhysicalDomain=network_engine_domain  SubClassName=ps_output  LeftPortType=input  RightPortType=output  PseudoPeriodic=off  Frequencies=[]  VectorFormat=1-D array  Unit=inherit  AffineConversion=off
  RHonClubFGlobal : Product  Multiplication=Matrix(*)
  RHonClubTGlobal : Product  Multiplication=Matrix(*)
  RW Kinematically Driven : Subsystem  Commented=on
  RW Kinetically Driven : Subsystem
  RWGlobalPosition : nesl_utility/PS-Simulink Converter  PhysicalDomain=network_engine_domain  SubClassName=ps_output  LeftPortType=input  RightPortType=output  PseudoPeriodic=off  Frequencies=[]  VectorFormat=1-D array  Unit=inherit  AffineConversion=off
  RWonRHFGlobal : Product  Multiplication=Matrix(*)
  RWonRHTGlobal : Product  Multiplication=Matrix(*)
  RightHandGlobaPosition : nesl_utility/PS-Simulink Converter  PhysicalDomain=network_engine_domain  SubClassName=ps_output  LeftPortType=input  RightPortType=output  PseudoPeriodic=off  Frequencies=[]  VectorFormat=1-D array  Unit=inherit  AffineConversion=off
  RotationMatrix : nesl_utility/PS-Simulink Converter  PhysicalDomain=network_engine_domain  SubClassName=ps_output  LeftPortType=input  RightPortType=output  PseudoPeriodic=off  Frequencies=[]  VectorFormat=1-D array  Unit=inherit  AffineConversion=off
  RotationMatrixRW : nesl_utility/PS-Simulink Converter  PhysicalDomain=network_engine_domain  SubClassName=ps_output  LeftPortType=input  RightPortType=output  PseudoPeriodic=off  Frequencies=[]  VectorFormat=1-D array  Unit=inherit  AffineConversion=off
  Transform Sensor1 : sm_lib/Frames and Transforms/Transform Sensor  MeasurementFrame=World  RotationSequence=XYX  SenseAngle=off  SenseAxis=off  SenseQ=off  SenseR=on  SenseRotationSequence=off  SenseOmegaX=off  SenseOmegaY=off  SenseOmegaZ=off  SenseOmega=off  SenseQDot=off  SenseRDot=off  SenseRotationSequenceDot=off  SenseAlphaX=off  SenseAlphaY=off  SenseAlphaZ=off  SenseAlpha=off  SenseQDDot=off  SenseRDDot=off  SenseX=off  SenseY=off  SenseZ=off  SenseXYZ=on  SenseRad=off  SenseAzim=off  SenseDist=off  SenseInc=off  SenseXDot=off  SenseYDot=off  SenseZDot=off  SenseXYZDot=off  SenseRadDot=off  SenseAzimDot=off  SenseDistDot=off  SenseIncDot=off  SenseXDDot=off  SenseYDDot=off  SenseZDDot=off  SenseXYZDDot=off  SenseRadDDot=off  SenseAzimDDot=off  SenseDistDDot=off  SenseIncDDot=off
  Transform Sensor2 : sm_lib/Frames and Transforms/Transform Sensor  MeasurementFrame=World  RotationSequence=XYX  SenseAngle=off  SenseAxis=off  SenseQ=off  SenseR=on  SenseRotationSequence=off  SenseOmegaX=off  SenseOmegaY=off  SenseOmegaZ=off  SenseOmega=off  SenseQDot=off  SenseRDot=off  SenseRotationSequenceDot=off  SenseAlphaX=off  SenseAlphaY=off  SenseAlphaZ=off  SenseAlpha=off  SenseQDDot=off  SenseRDDot=off  SenseX=off  SenseY=off  SenseZ=off  SenseXYZ=on  SenseRad=off  SenseAzim=off  SenseDist=off  SenseInc=off  SenseXDot=off  SenseYDot=off  SenseZDot=off  SenseXYZDot=off  SenseRadDot=off  SenseAzimDot=off  SenseDistDot=off  SenseIncDot=off  SenseXDDot=off  SenseYDDot=off  SenseZDDot=off  SenseXYZDDot=off  SenseRadDDot=off  SenseAzimDDot=off  SenseDistDDot=off  SenseIncDDot=off
  Transform Sensor4 : sm_lib/Frames and Transforms/Transform Sensor  MeasurementFrame=World  RotationSequence=XYX  SenseAngle=off  SenseAxis=off  SenseQ=off  SenseR=on  SenseRotationSequence=off  SenseOmegaX=off  SenseOmegaY=off  SenseOmegaZ=off  SenseOmega=off  SenseQDot=off  SenseRDot=off  SenseRotationSequenceDot=off  SenseAlphaX=off  SenseAlphaY=off  SenseAlphaZ=off  SenseAlpha=off  SenseQDDot=off  SenseRDDot=off  SenseX=off  SenseY=off  SenseZ=off  SenseXYZ=off  SenseRad=off  SenseAzim=off  SenseDist=off  SenseInc=off  SenseXDot=off  SenseYDot=off  SenseZDot=off  SenseXYZDot=off  SenseRadDot=off  SenseAzimDot=off  SenseDistDot=off  SenseIncDot=off  SenseXDDot=off  SenseYDDot=off  SenseZDDot=off  SenseXYZDDot=off  SenseRadDDot=off  SenseAzimDDot=off  SenseDistDDot=off  SenseIncDDot=off
  World Frame1 : sm_lib/Frames and Transforms/World Frame
  World Frame2 : sm_lib/Frames and Transforms/World Frame
  Bottom of Right Forearm : PMIOPort  Side=Left
  RHandLocationonClub : PMIOPort  Port=2  Side=Right
  RH GripStandoff : PMIOPort  Port=3  Side=Right
  tag scope: RHGlobalPosition=global, RHonClubFGlobalOut=global, RHonClubTGlobalOut=global, RWGlobalPosition=global, RWLocaltoGlobalR=global, RWTorqueGlobal=global, RWonRHFGlobalOut=global, RWonRHTGlobalOut=global
  wires:
  [RHonClubForceLocal] -> RHonClubFGlobal/2
  RotationMatrix/1 -> RHonClubTGlobal/1, RHonClubFGlobal/1
  RHonClubFGlobal/1 -> [RHonClubFGlobalOut]  "RHonClubFGlobal"
  RHonClubTGlobal/1 -> [RHonClubTGlobalOut]  "RHonClubTGlobal"
  [RHonClubTorqueLocal] -> RHonClubTGlobal/2
  RWonRHTGlobal/1 -> [RWonRHTGlobalOut]  "RWonRHTGlobal"
  RotationMatrixRW/1 -> RWonRHTGlobal/1, RWonRHFGlobal/1
  RWGlobalPosition/1 -> [RWGlobalPosition]  "RWGlobalPosition"
  RWonRHFGlobal/1 -> [RWonRHFGlobalOut]  "RWonRHFGlobal"
  RightHandGlobaPosition/1 -> [RHGlobalPosition]  "RHGlobalPosition"
  [RWForceLocal] -> RWonRHFGlobal/2
  [RWTorqueLocal] -> RWonRHTGlobal/2
  PS-Simulink Converter1/1 -> [RWLocaltoGlobalR], Matrix Multiply/1
  Matrix Multiply/1 -> [RWTorqueGlobal]  "RWTorqueGlobal"
  [RWTorqueLocal] -> Matrix Multiply/2
  connections:
  RotationMatrix/LConn1 -- Transform Sensor1/RConn2
  World Frame1/RConn1 -- Transform Sensor4/LConn1 -- Transform Sensor1/LConn1
  Transform Sensor1/RConn3 -- RightHandGlobaPosition/LConn1
  RHandLocationonClub/RConn1 -- Transform Sensor1/RConn1
  RotationMatrixRW/LConn1 -- Transform Sensor2/RConn2
  World Frame2/RConn1 -- Transform Sensor2/LConn1
  Transform Sensor2/RConn3 -- RWGlobalPosition/LConn1
  Transform Sensor2/RConn1 -- Transform Sensor4/RConn1 -- RW Kinematically Driven/RConn1 -- RH GripStandoff/RConn1 -- RW Kinetically Driven/RConn1
  RW Kinetically Driven/LConn1 -- RW Kinematically Driven/LConn1 -- Bottom of Right Forearm/RConn1
  Transform Sensor4/RConn2 -- PS-Simulink Converter1/LConn1
